simulink model "codegen_drive_manual"  (R2025b)
settings: Solver=FixedStepAuto  StartTime=0.0  StopTime=10.0  FixedStep=0.001  RelTol=1e-3
settings Model: Creator=rowan  LastModifiedBy=rowan
settings OptimizationCC: DefaultParameterBehavior=Inlined  UseDivisionForNetSlopeComputation=on  GainParamInheritBuiltInType=on  UseFloatMulNetSlope=on  InlineInvariantSignals=on  PassReuseOutputArgsAs=Individual arguments  ZeroExternalMemoryAtStartup=off  ZeroInternalMemoryAtStartup=off  NoFixptDivByZeroProtection=on  EfficientFloat2IntCast=on  LifeSpan=1  OptimizeBlockOrder=speed  DifferentSizesBufferReuse=on  EfficientTunableParamExpr=on
settings DebuggingCC: ParameterTunabilityLossMsg=error
settings HardwareCC: ProdBitPerInt=16.0  ProdBitPerPointer=16.0  ProdBitPerSizeT=16.0  ProdBitPerPtrDiffT=16.0  ProdLargestAtomicFloat=None  ProdWordSize=16.0  ProdLongLongMode=on  ProdHWDeviceType=STMicroelectronics->ST10/Super10
settings SFSimCC: MATLABDynamicMemAlloc=off
settings RTWCC: SystemTargetFile=ert.tlc  TemplateMakefile=ert_default_tmf  Description=Embedded Coder
settings CodeAppCC: ForceParamTrailComments=on  IgnoreCustomStorageClasses=off  OperatorAnnotations=on  SimulinkDataObjDesc=on  SFDataObjDesc=on  CustomSymbolStrGlobalVar=rt$N$M  CustomSymbolStrType=$N$M  CustomSymbolStrFcn=$N$M$F  CustomSymbolStrMacro=$N$M  InsertBlockDesc=on
settings ERTTargetCC: ERTCustomFileTemplate=example_file_process.tlc  ERTFilePackagingFormat=CompactWithDataFile  TargetLangStandard=C99 (ISO)  GenerateSampleERTMain=on  IncludeMdlTerminateFcn=off  CombineSignalStateStructs=on  SupportAbsoluteTime=off  SupportComplex=off  SupportNonInlinedSFcns=on

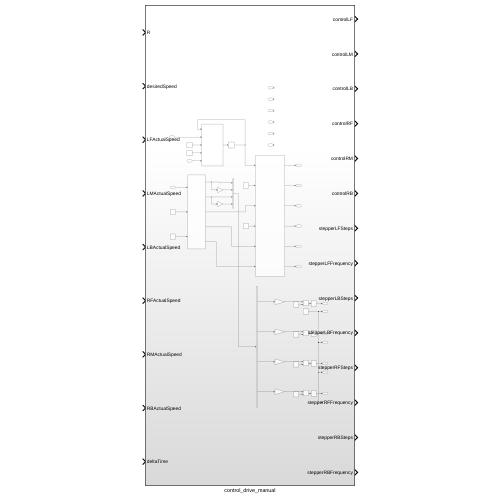
[thumbnail: Simulink's stored preview of the top-level diagram]
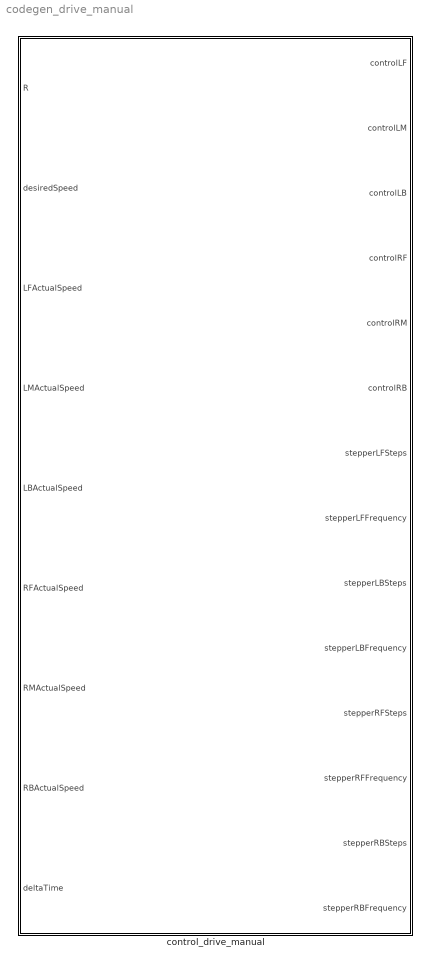
== system codegen_drive_manual ==
  control_drive_manual : Subsystem

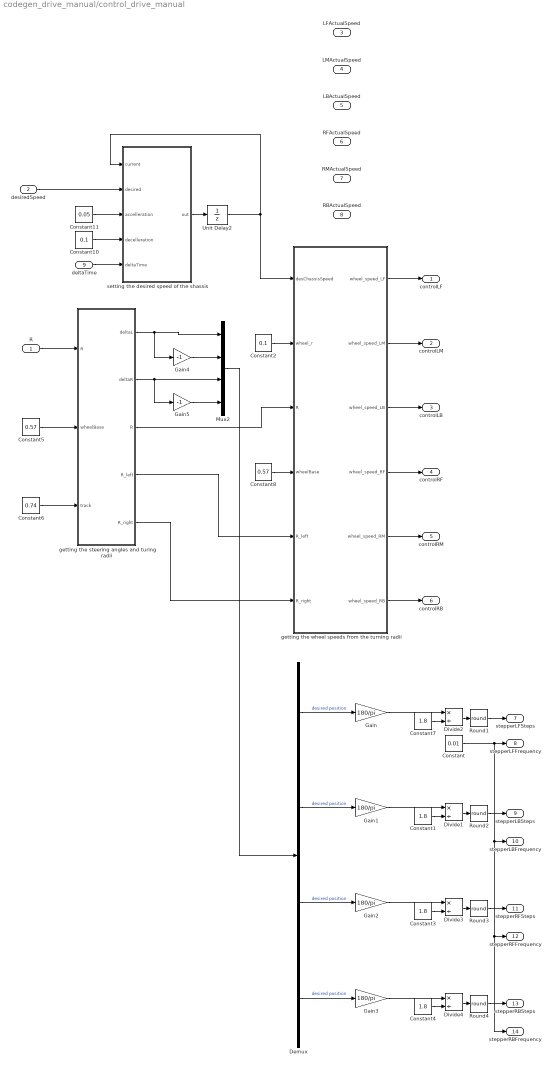
== system codegen_drive_manual/control_drive_manual ==
  R : Inport
  desiredSpeed : Inport  Port=2
  LFActualSpeed : Inport  Port=3
  LMActualSpeed : Inport  Port=4
  LBActualSpeed : Inport  Port=5
  RFActualSpeed : Inport  Port=6
  RMActualSpeed : Inport  Port=7
  RBActualSpeed : Inport  Port=8
  deltaTime : Inport  Port=9
  Constant : Constant  Value=0.01
  Constant{1,3..4,7} (4 alike) : Constant  Value=1.8
  Constant10 : Constant  Value=0.1
  Constant11 : Constant  Value=0.05
  Constant2 : Constant  Value=0.1
  Constant5 : Constant  Value=0.57
  Constant6 : Constant  Value=0.74
  Constant8 : Constant  Value=0.57
  Demux : Demux
  Divide{1..4} (4 alike) : Product  Inputs=*/
  Gain{,1..3} (4 alike) : Gain  Gain=180/pi
  Gain4 : Gain  Gain=-1
  Gain5 : Gain  Gain=-1
  Mux2 : Mux
  Round{1..4} (4 alike) : Rounding  Operator=round
  Unit Delay2 : UnitDelay  SampleTime=-1  HasFrameUpgradeWarning=on
  getting the steering angles and turing radii : MATLAB Function  TreatAsAtomicUnit=on
  getting the wheel speeds from the turning radii : MATLAB Function  TreatAsAtomicUnit=on
  setting the desired speed of the shassis : MATLAB Function  TreatAsAtomicUnit=on
  controlLF : Outport
  controlLM : Outport  Port=2
  controlLB : Outport  Port=3
  controlRF : Outport  Port=4
  controlRM : Outport  Port=5
  controlRB : Outport  Port=6
  stepperLFSteps : Outport  Port=7
  stepperLFFrequency : Outport  Port=8
  stepperLBSteps : Outport  Port=9
  stepperLBFrequency : Outport  Port=10
  stepperRFSteps : Outport  Port=11
  stepperRFFrequency : Outport  Port=12
  stepperRBSteps : Outport  Port=13
  stepperRBFrequency : Outport  Port=14
  wires:
  Mux2/1 -> Demux/1
  desiredSpeed/1 -> setting the desired speed of the shassis/2(desired)
  Unit Delay2/1 -> setting the desired speed of the shassis/1(current), getting the wheel speeds from the turning radii/1(desChassisSpeed)
  getting the steering angles and turing radii/5(R_right) -> getting the wheel speeds from the turning radii/6(R_right)
  getting the steering angles and turing radii/1(deltaL) -> Mux2/1, Gain4/1
  Gain4/1 -> Mux2/2
  getting the steering angles and turing radii/4(R_left) -> getting the wheel speeds from the turning radii/5(R_left)
  getting the steering angles and turing radii/2(deltaR) -> Mux2/3, Gain5/1
  Gain5/1 -> Mux2/4
  getting the steering angles and turing radii/3(R) -> getting the wheel speeds from the turning radii/3(R)
  Constant2/1 -> getting the wheel speeds from the turning radii/2(wheel_r)
  R/1 -> getting the steering angles and turing radii/1("R ")
  Demux/1 -> Gain/1  "desired position"
  Constant7/1 -> Divide2/2
  Divide2/1 -> Round1/1
  Round1/1 -> stepperLFSteps/1
  Divide1/1 -> Round2/1
  Constant1/1 -> Divide1/2
  Demux/2 -> Gain1/1  "desired position"
  Round2/1 -> stepperLBSteps/1
  Divide3/1 -> Round3/1
  Constant3/1 -> Divide3/2
  Demux/3 -> Gain2/1  "desired position"
  Round3/1 -> stepperRFSteps/1
  Divide4/1 -> Round4/1
  Constant4/1 -> Divide4/2
  Demux/4 -> Gain3/1  "desired position"
  Round4/1 -> stepperRBSteps/1
  Constant/1 -> stepperLFFrequency/1, stepperRBFrequency/1, stepperRFFrequency/1, stepperLBFrequency/1
  Gain/1 -> Divide2/1
  Gain1/1 -> Divide1/1
  Gain2/1 -> Divide3/1
  Gain3/1 -> Divide4/1
  Constant6/1 -> getting the steering angles and turing radii/3(track)
  Constant5/1 -> getting the steering angles and turing radii/2(wheelBase)
  Constant8/1 -> getting the wheel speeds from the turning radii/4(wheelBase)
  setting the desired speed of the shassis/1(out) -> Unit Delay2/1
  getting the wheel speeds from the turning radii/1(wheel_speed_LF) -> controlLF/1
  getting the wheel speeds from the turning radii/2(wheel_speed_LM) -> controlLM/1
  getting the wheel speeds from the turning radii/3(wheel_speed_LB) -> controlLB/1
  getting the wheel speeds from the turning radii/4(wheel_speed_RF) -> controlRF/1
  getting the wheel speeds from the turning radii/5(wheel_speed_RM) -> controlRM/1
  getting the wheel speeds from the turning radii/6(wheel_speed_RB) -> controlRB/1
  Constant11/1 -> setting the desired speed of the shassis/3(accelleration)
  Constant10/1 -> setting the desired speed of the shassis/4(decelleration)
  deltaTime/1 -> setting the desired speed of the shassis/5(deltaTime)

== matlab function codegen_drive_manual/control_drive_manual/getting the wheel speeds from the turning radii ==
  data: desChassisSpeed input; wheel_speed_LF output; wheel_r input; R input; wheelBase input; R_left input; R_right input; wheel_speed_LM output; wheel_speed_LB output; wheel_speed_RF output; wheel_speed_RM output; wheel_speed_RB output
function [wheel_speed_LF,wheel_speed_LM,wheel_speed_LB,wheel_speed_RF,wheel_speed_RM,wheel_speed_RB] = ...
          ackermann_speeds(desChassisSpeed,wheel_r,R,wheelBase,R_left,R_right)

gearRatio = 10;

if R > 0
    wheel_speed_LF = (desChassisSpeed/wheel_r)*sqrt(R_left^2 + (wheelBase/2)^2)/R;
    wheel_speed_LM = desChassisSpeed * R_left/(R*wheel_r);
    wheel_speed_LB = (desChassisSpeed/wheel_r)*sqrt(R_left^2 + (wheelBase/2)^2)/R;
    wheel_speed_RF = (desChassisSpeed/wheel_r)*sqrt(R_right^2 + (wheelBase/2)^2)/R;
    wheel_speed_RM = desChassisSpeed * R_right/(R*wheel_r);
    wheel_speed_RB = (desChassisSpeed/wheel_r)*sqrt(R_right^2 + (wheelBase/2)^2)/R;
else
    wheel_speed_LF = desChassisSpeed / wheel_r;
    wheel_speed_LM = desChassisSpeed / wheel_r;
    wheel_speed_LB = desChassisSpeed / wheel_r;
    wheel_speed_RF = desChassisSpeed / wheel_r;
    wheel_speed_RM = desChassisSpeed / wheel_r;
    wheel_speed_RB = desChassisSpeed / wheel_r;
end
%{
    wheel_speed_LF = wheel_speed_LF * gearRatio;
    wheel_speed_LM = wheel_speed_LM * gearRatio;
    wheel_speed_LB = wheel_speed_LB * gearRatio;
    wheel_speed_RF = wheel_speed_RF * gearRatio;
    wheel_speed_RM = wheel_speed_RM * gearRatio;
    wheel_speed_RB = wheel_speed_RB * gearRatio;
%}
end

== matlab function codegen_drive_manual/control_drive_manual/getting the steering angles and turing radii ==
  data: R input; deltaL output; deltaR output; R output; R_left output; R_right output; wheelBase input; track input
function [deltaL,deltaR,R,R_left,R_right] = ackermann_angles(R,wheelBase,track)
    % Function to compute ackerman steering angles
    if R < 0
        R_left = (R+track/2);
        R_right = (R-track/2);
        deltaL = atan(wheelBase/(R_left));
        deltaR = atan(wheelBase/(R_right));
    elseif R > 0
        R_left = (R-track/2);
        R_right = (R+track/2);
        deltaL = -atan(wheelBase/(R_left));
        deltaR = -atan(wheelBase/(R_right));
    else
        deltaL = 0;
        deltaR = 0;
        R_left = R;
        R_right = R;
    end
    R = abs(R);
end

== matlab function codegen_drive_manual/control_drive_manual/setting the desired speed of the shassis ==
  data: current input; out output; desired input; accelleration input; decelleration input; deltaTime input
function out = linear_interpolation(current, desired, accelleration, decelleration, deltaTime)
%accellerating slower than decellerating
if current >= 0
    if current < desired
        current = current + accelleration * deltaTime;
    end
    if current > desired
        current = current - decelleration * deltaTime;
    end
end
%doing the same going backwards
if current <= 0
    if current > desired
        current = current - accelleration * deltaTime;
    end
    if current < desired
        current = current + decelleration * deltaTime;
    end
end
out = current;
